simulink model "motor_driver"  (R2017b)
settings: Solver=ode3  StartTime=0.0  StopTime=0.5  FixedStep=0.0002  RelTol=1e-3
libraries: stellaris_lp_lib x4, simulink x3
settings Model: ExtModeTrigDuration=2  Creator=peselnikmg  LastModifiedBy=Joshua
settings DataIOCC: LimitDataPoints=on  SaveFormat=Array  SignalLoggingSaveFormat=ModelDataLogs
settings OptimizationCC: PassReuseOutputArgsAs=Individual arguments  ExpressionDepthLimit=2147483647  MaxStackSize=64
settings DebuggingCC: ParameterTunabilityLossMsg=error  StateNameClashWarn=warning  SFUnexpectedBacktrackingDiag=warning  SFNoUnconditionalDefaultTransitionDiag=warning  SFExecutionAtInitializationDiag=none
settings HardwareCC: ProdBitPerPointer=32  ProdBitPerSizeT=32  ProdBitPerPtrDiffT=32  ProdLargestAtomicInteger=Long  ProdLargestAtomicFloat=Double  ProdWordSize=32  ProdHWDeviceType=ARM Compatible->ARM Cortex
settings ModelReferenceCC: PropagateSignalLabelsOutOfModel=off
settings SFSimCC: MATLABDynamicMemAlloc=off
settings RTWCC: SystemTargetFile=ert.tlc  HardwareBoard=Tiva TM4C123G Launchpad  TLCOptions=-aInlineSetEventsForThisBaseRateFcn=TLC_FALSE -aSuppressMultiTaskScheduler=TLC_FALSE -aRateBasedStepFcn=1  TemplateMakefile=ert_default_tmf  GenerateReport=on  RTWVerbose=off  Toolchain=Texas Instruments Code Composer Studio (Tiva)  IncludeHyperlinkInReport=on  LaunchReport=on  GenerateTraceInfo=on  GenerateTraceReport=on  GenerateTraceReportSl=on  GenerateTraceReportSf=on  GenerateTraceReportEml=on
settings CodeAppCC: ForceParamTrailComments=on  IgnoreCustomStorageClasses=off  OperatorAnnotations=on  SimulinkDataObjDesc=on  SFDataObjDesc=on  MATLABFcnDesc=on  CustomSymbolStrType=$N$R$M  InsertBlockDesc=on  StateflowObjectComments=on  MATLABSourceComments=on  InternalIdentifier=Classic
settings ConfigComp: CovMetricSettings=dw  CovHtmlReporting=on  CovSaveCumulativeToWorkspaceVar=on  CovSaveSingleToWorkspaceVar=on  CovExternalEMLEnable=off
settings SimscapeCC: SimscapeNormalizeSystem=off

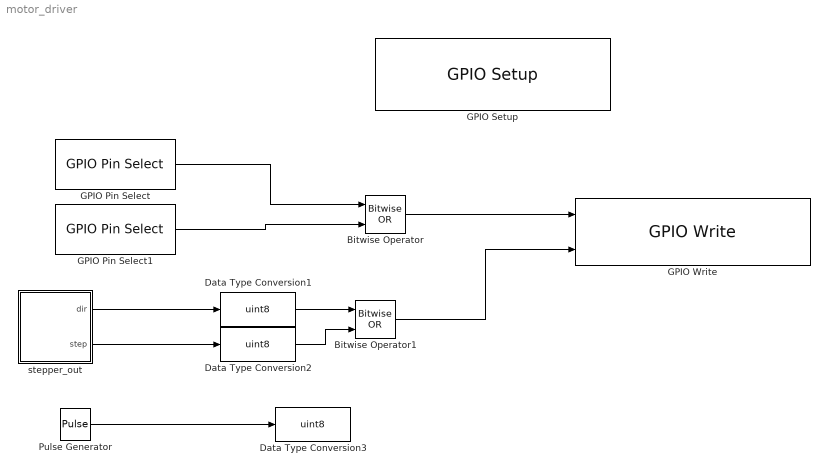
== system motor_driver ==
  Bitwise Operator : simulink/Logic and Bit Operations/Bitwise Operator  logicop=OR  UseBitMask=off  NumInputPorts=2  BitMask=bin2dec('11011001')  BitMaskRealWorld=Stored Integer
  Bitwise Operator1 : simulink/Logic and Bit Operations/Bitwise Operator  logicop=OR  UseBitMask=off  NumInputPorts=2  BitMask=bin2dec('11011001')  BitMaskRealWorld=Stored Integer
  Data Type Conversion1 : DataTypeConversion  OutDataTypeStr=uint8
  Data Type Conversion2 : DataTypeConversion  OutDataTypeStr=uint8
  Data Type Conversion3 : DataTypeConversion  OutDataTypeStr=uint8
  GPIO Pin Select : stellaris_lp_lib/GPIO/GPIO Pin Select  GPIO_PIN_X=GPIO_PIN_2
      settings: SourceProductName=Run on Stellaris LaunchPad
  GPIO Pin Select1 : stellaris_lp_lib/GPIO/GPIO Pin Select  GPIO_PIN_X=GPIO_PIN_3
      settings: SourceProductName=Run on Stellaris LaunchPad
  GPIO Setup : stellaris_lp_lib/GPIO/GPIO Setup  GPIO_PORTX_BASE=GPIO_PORTF_BASE  PinsOutput_0=Unused  PinsOutput_1=Unused  PinsOutput_2=Output  PinsOutput_3=Output  PinsOutput_4=Unused  PinsOutput_5=Unused  PinsOutput_6=Unused  PinsOutput_7=Unused
      settings: SourceProductName=Run on Stellaris LaunchPad
  GPIO Write : stellaris_lp_lib/GPIO/GPIO Write  GPIO_PORTX_BASE=GPIO_PORTF_BASE  SampleTime=-1
      settings: SourceProductName=Run on Stellaris LaunchPad
  Pulse Generator : DiscretePulseGenerator  PulseType=Time based  Amplitude=15  Period=0.002  PulseWidth=50
  stepper_out : Subsystem
  wires:
  Bitwise Operator/1 -> GPIO Write/1
  GPIO Pin Select/1 -> Bitwise Operator/1
  GPIO Pin Select1/1 -> Bitwise Operator/2
  stepper_out/1(dir) -> Data Type Conversion1/1
  Data Type Conversion1/1 -> Bitwise Operator1/1
  stepper_out/2(step) -> Data Type Conversion2/1
  Data Type Conversion2/1 -> Bitwise Operator1/2
  Pulse Generator/1 -> Data Type Conversion3/1
  Bitwise Operator1/1 -> GPIO Write/2

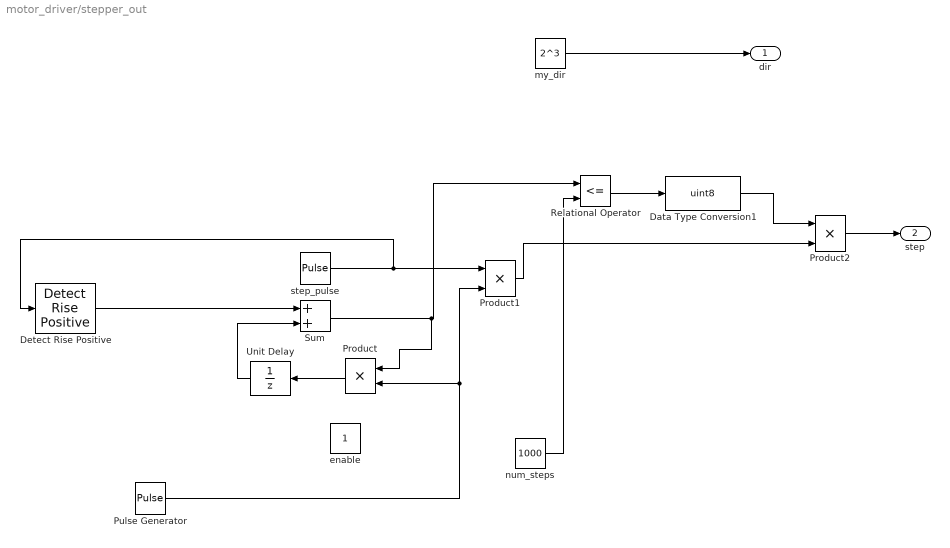
== system motor_driver/stepper_out ==
  Data Type Conversion1 : DataTypeConversion  OutDataTypeStr=uint8
  Detect Rise Positive : simulink/Logic and Bit Operations/Detect Rise Positive  vinit=0  OutDataTypeStr=boolean
  Product : Product  OutDataTypeStr=uint32
  Product1 : Product  OutDataTypeStr=uint8
  Product2 : Product  OutDataTypeStr=uint8
  Pulse Generator : DiscretePulseGenerator  PulseType=Time based  Period=5  PulseWidth=90
  Relational Operator : RelationalOperator  Operator=<=  OutDataTypeStr=boolean  RndMeth=Simplest
  Sum : Sum  AccumDataTypeStr=uint32  OutDataTypeStr=uint32  SaturateOnIntegerOverflow=on
  Unit Delay : UnitDelay  SampleTime=-1
  enable : Constant  OutDataTypeStr=uint8
  my_dir : Constant  Value=2^3  OutDataTypeStr=uint8
  num_steps : Constant  Value=1000  OutDataTypeStr=uint32
  step_pulse : DiscretePulseGenerator  PulseType=Time based  Amplitude=2^2  Period=0.002  PulseWidth=50
  dir : Outport
  step : Outport  Port=2
  wires:
  Product/1 -> Unit Delay/1
  Unit Delay/1 -> Sum/2
  step_pulse/1 -> Product1/1, Detect Rise Positive/1
  Product2/1 -> step/1
  Product1/1 -> Product2/2
  Relational Operator/1 -> Data Type Conversion1/1
  Data Type Conversion1/1 -> Product2/1
  Detect Rise Positive/1 -> Sum/1
  Pulse Generator/1 -> Product/2, Product1/2
  num_steps/1 -> Relational Operator/2
  Sum/1 -> Product/1, Relational Operator/1
  my_dir/1 -> dir/1
